simulink model "DiscreteStateSpace_TestGen5"  (R2017b)
settings: Solver=FixedStepDiscrete  StartTime=0.0  StopTime=10.0  RelTol=1e-3
settings Model: Creator=ktrinh  LastModifiedBy=ktrinh
settings DebuggingCC: ParameterOverflowMsg=none

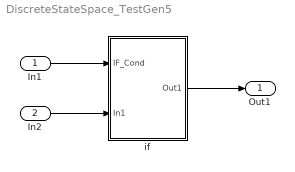
== system DiscreteStateSpace_TestGen5 ==
  In1 : Inport
  In2 : Inport  Port=2
  if : Subsystem  AncestorBlock=Block_TestLib/if
  Out1 : Outport
  wires:
  In1/1 -> if/1(IF_Cond)
  In2/1 -> if/2(In1)
  if/1(Out1) -> Out1/1

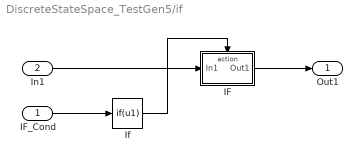
== system DiscreteStateSpace_TestGen5/if ==
  IF_Cond : Inport  OutDataTypeStr=boolean
  In1 : Inport  Port=2
  IF : Subsystem  TreatAsAtomicUnit=on
  If : If  IfExpression=u1  ShowElse=off
  Out1 : Outport
  wires:
  If/1 -> IF/Action
  In1/1 -> IF/1(In1)
  IF_Cond/1 -> If/1
  IF/1(Out1) -> Out1/1

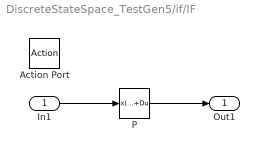
== system DiscreteStateSpace_TestGen5/if/IF ==
  In1 : Inport
  Action Port : ActionPort  ActionType=then
  P : DiscreteStateSpace  A=[0.5 0.6;0.7 0.8]  B=[1;0.2]  C=[0.5 1]  SampleTime=-1
  Out1 : Outport
  wires:
  In1/1 -> P/1
  P/1 -> Out1/1
